simulink model "Junctions2NoActions"  (Simulink 9.0)
settings: Solver=FixedStepDiscrete  StartTime=0.0  StopTime=10.0  RelTol=1e-3  EnableMultiTasking=on
model workspace (MAT data in the model file):
  x3 = Simulink.Parameter
  x3.Value = 333
  x3.DataType = 'int32'
  x3.Dimensions = [1 1]
  x4 = Simulink.Parameter
  x4.Value = 542
  x4.DataType = 'double'
  x4.Dimensions = [1 1]
settings Model: SuppressorTable=22 serialization::archive 11 0 6 0 0 0 0 0  Creator=scaife  LastModifiedBy=ktrinh  ExtModeAutoUpdateStatusClock=off
settings DataIOCC: LimitDataPoints=on  SignalLoggingSaveFormat=ModelDataLogs  SignalLoggingName=sigsOut
settings DebuggingCC: SaveWithParameterizedLinksMsg=none  SignalResolutionControl=TryResolveAllWithWarning  MultiTaskDSMMsg=warning  MultiTaskCondExecSysMsg=none
settings HardwareCC: TargetUnknown=on
settings SFSimCC: SimParseCustomCode=off
settings GRTTargetCC: GeneratePreprocessorConditionals=Disable all  CombineOutputUpdateFcns=off  GRTInterface=on

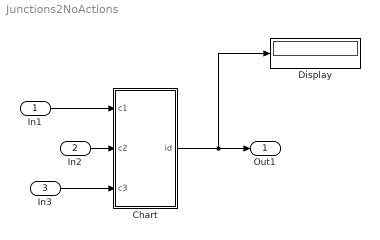
== system Junctions2NoActions ==
  In1 : Inport  OutDataTypeStr=boolean
  In2 : Inport  Port=2  OutDataTypeStr=boolean
  In3 : Inport  Port=3  OutDataTypeStr=boolean
  Chart : Stateflow chart  TreatAsAtomicUnit=on
  Display : Display
  Out1 : Outport
  wires:
  Chart/1(id) -> Out1/1, Display/1
  In1/1 -> Chart/1(c1)
  In2/1 -> Chart/2(c2)
  In3/1 -> Chart/3(c3)

== stateflow chart Chart ==
  state A
    en: id=1;
  state C
    en: id=4;
  state B
    en: id = 2;
  state D
    en: id = 3;
  (junction 12) -> (junction 11) [order 3]
  (default) -> A
  A -> (junction 12) [order 1] : [c1]
  (junction 12) -> B [order 1] : [c2]
  (junction 12) -> D [order 2] : [c3]
  A -> C [order 2] : [c1]
  data: c1 input double; c2 input double; c3 input double; id output double
